simulink model "L22B2"  (R2015a)
settings: Solver=ode45  StartTime=0.0  StopTime=1  RelTol=1e-3
values from neighbouring files (symbols this model uses):
  a1 = ke*km/J/La    (= 10740.9160847)    [L22m.m]
  a2 = Ra/La    (= 294.117647059)    [L22m.m]
  b = -km*kp/J/La    (= -1139188.06959)    [L22m.m]
  c = 10000    [L22m.m]
  deltaB2 = 0.2    [L22m.m]
  fmaxB2 = 1e+7    (= 10000000)    [L22m.m]
  J = 0.71e-3    (= 0.00071)    [L22m.m]
  ke = 0.33    [L22m.m]
  km = ke    (= 0.33)    [L22m.m]
  kp = 35    [L22m.m]
  La = 14.28e-3    (= 0.01428)    [L22m.m]
  Ra = 4.2    [L22m.m]
  v = -12    [L22m.m]
  vTime = 0.6    [L22m.m]
  w = 20    [L22m.m]
settings Model: Creator=B014-5  LastModifiedBy=B014-5

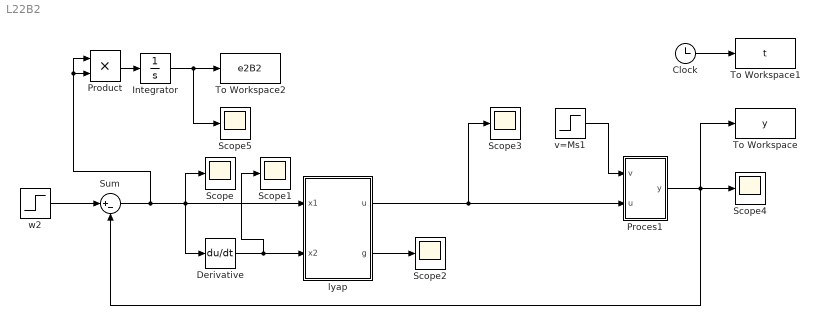
== system L22B2 ==
  Clock : Clock
  Derivative : Derivative
  Integrator : Integrator
  Proces1 : Subsystem
  Product : Product
  Scope{,1..5} (6 alike) : Scope
      Scope1 settings: SaveName=ScopeData2
      Scope2 settings: SaveName=ScopeData3
      Scope3 settings: SaveName=ScopeData4
      Scope4 settings: YMin=0  YMax=21  SaveName=ScopeData5
  Sum : Sum  Inputs=|+-
  To Workspace : ToWorkspace  VariableName=y  SampleTime=-1
  To Workspace1 : ToWorkspace  VariableName=t  SampleTime=-1
  To Workspace2 : ToWorkspace  VariableName=e2B2  SampleTime=-1
  lyap : Subsystem
  v=Ms1 : Step  Time=vTime  After=v  SampleTime=0
  w2 : Step  Time=0  After=w  SampleTime=0
  wires:
  w2/1 -> Sum/1
  Sum/1 -> Product/1, Product/2, Derivative/1, lyap/1(x1), Scope/1
  Derivative/1 -> Scope1/1, lyap/2(x2)
  lyap/2(g) -> Scope2/1
  lyap/1(u) -> Proces1/2(u), Scope3/1
  v=Ms1/1 -> Proces1/1(v)
  Proces1/1(y) -> To Workspace/1, Sum/2, Scope4/1
  Clock/1 -> To Workspace1/1
  Product/1 -> Integrator/1
  Integrator/1 -> Scope5/1, To Workspace2/1

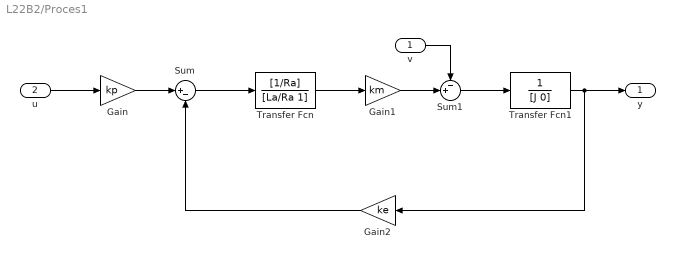
== system L22B2/Proces1 ==
  v : Inport
  u : Inport  Port=2
  Gain : Gain  Gain=kp
  Gain1 : Gain  Gain=km
  Gain2 : Gain  Gain=ke
  Sum : Sum  Inputs=|+-
  Sum1 : Sum  Inputs=-+|
  Transfer Fcn : TransferFcn  Numerator=[1/Ra]  Denominator=[La/Ra 1]
  Transfer Fcn1 : TransferFcn  Denominator=[J 0]
  y : Outport
  wires:
  v/1 -> Sum1/1
  Gain/1 -> Sum/1
  Transfer Fcn1/1 -> y/1, Gain2/1
  Sum1/1 -> Transfer Fcn1/1
  Sum/1 -> Transfer Fcn/1
  Gain2/1 -> Sum/2
  u/1 -> Gain/1
  Gain1/1 -> Sum1/2
  Transfer Fcn/1 -> Gain1/1

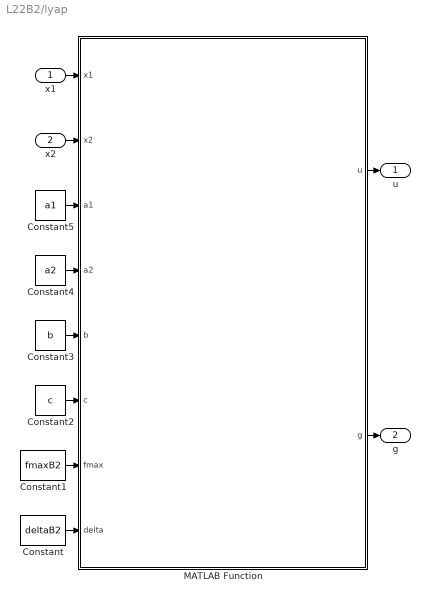
== system L22B2/lyap ==
  x1 : Inport
  x2 : Inport  Port=2
  Constant : Constant  Value=deltaB2
  Constant1 : Constant  Value=fmaxB2
  Constant2 : Constant  Value=c
  Constant3 : Constant  Value=b
  Constant4 : Constant  Value=a2
  Constant5 : Constant  Value=a1
  MATLAB Function : MATLAB Function  TreatAsAtomicUnit=on
  u : Outport
  g : Outport  Port=2
  wires:
  Constant2/1 -> MATLAB Function/6(c)
  Constant5/1 -> MATLAB Function/3(a1)
  Constant1/1 -> MATLAB Function/7(fmax)
  Constant4/1 -> MATLAB Function/4(a2)
  x2/1 -> MATLAB Function/2(x2)
  MATLAB Function/2(g) -> g/1
  Constant/1 -> MATLAB Function/8(delta)
  MATLAB Function/1(u) -> u/1
  x1/1 -> MATLAB Function/1(x1)
  Constant3/1 -> MATLAB Function/5(b)

== matlab function L22B2/lyap/MATLAB Function ==
  data: u output; g output; x1 input; x2 input; a1 input; a2 input; b input; c input; fmax input; delta input
function [u, g] = lyap(x1, x2, a1, a2, b, c, fmax, delta)
%#codegen

g = c * x1 + x2;
u = sign(g)*(abs((a1*x1-(c-a2)*x2)+fmax)/abs(b)+delta);
